simulink model "PFMODEL"  (R2023a)
settings: Solver=ode4  StartTime=0.0  StopTime=10  FixedStep=10e-6  RelTol=1e-3
libraries: spsPower3phInstantaneousLib x1, spsThreePhaseSeriesRLCLoadLib x1, spsThreePhaseVIMeasurementLib x1, spsThreePhaseSourceLib x1, sps_lib x1
settings Model: PacingRate=0.100000  Creator=KeronDenny  LastModifiedBy=KeronDenny

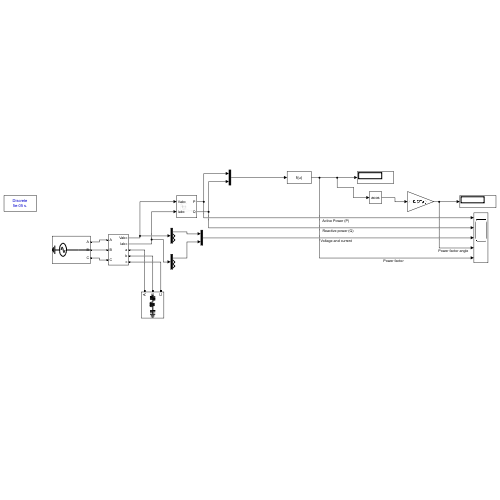
[thumbnail: Simulink's stored preview of the top-level diagram]
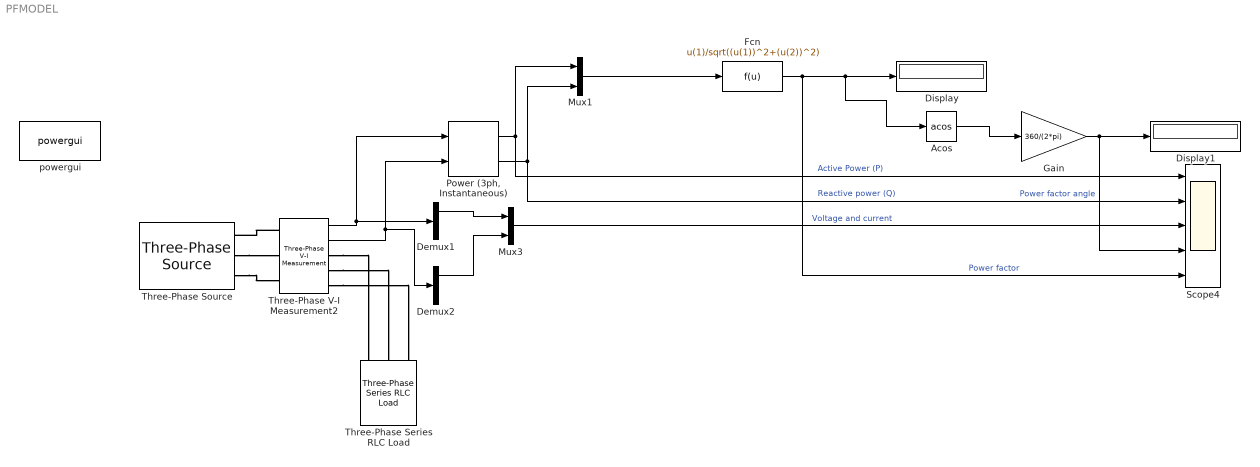
== system PFMODEL ==
  Acos : Trigonometry  Operator=acos
  Demux1 : Demux  Outputs=3
  Demux2 : Demux  Outputs=3
  Display : Display
  Display1 : Display
  Fcn : Fcn  Expr=u(1)/sqrt((u(1))^2+(u(2))^2)
  Gain : Gain  Gain=360/(2*pi)
  Mux1 : Mux  Inputs=2
  Mux3 : Mux  Inputs=2
  "Power (3ph, Instantaneous)" : spsPower3phInstantaneousLib/Power (3ph, Instantaneous)
  Scope4 : Scope  NumInputPorts=5
  Three-Phase Series RLC Load : spsThreePhaseSeriesRLCLoadLib/Three-Phase Series RLC Load  LConnTagsString=A|B|C  Configuration=Y (grounded)  NominalVoltage=400  Vabc=[1e3 1e3 1e3]  Vabcp=[1e3 1e3 1e3]  NominalFrequency=50  UnbalancedPower=off  ActivePower=40000  InductivePower=9012  CapacitivePower=35.92  Pabc=[10e3 9e3 11e3]  QLabc=[100 90 110]  QCabc=[100 90 110]  Pabcp=[10e3 9e3 11e3]  QLabcp=[100 90 110]  QCabcp=[100 90 110]  Measurements=None  LoadType=constant Z
  Three-Phase V-I Measurement2 : spsThreePhaseVIMeasurementLib/Three-Phase V-I Measurement  VoltageMeasurement=phase-to-ground  SetLabelV=off  LabelV=Vabc  Vpu=off  VpuLL=off  CurrentMeasurement=yes  SetLabelI=off  LabelI=Iabc  Ipu=off  Pbase=100e6  Vbase=500e3  OutputType=Complex  PhasorSimulation=off  PSBequivalent=0
  Three-Phase Source : spsThreePhaseSourceLib/Three-Phase Source  InternalConnection=Yg  VoltagePhases=off  Voltage=400  PhaseAngle=0  Voltage_phases=[25e3 25e3 25e3]/sqrt(3)  PhaseAngles_phases=[0 -120 +120]  Frequency=50  NonIdealSource=off  SpecifyImpedance=off  Resistance=0.8929  Inductance=16.58e-3  ShortCircuitLevel=100e6  BaseVoltage=25e3  XRratio=7  BusType=swing  Pref=10e3  Qref=0  Prefabc=[10e3, 10e3, 10e3]  Qrefabc=[0, 0, 0]  Qmin=-inf  Qmax=inf
  powergui : sps_lib/powergui  Priority=1  SimulationMode=Discrete  SampleTime=50e-6  frequency=60  Iterations=50  frequencyindice=50  Pbase=100e6  ErrMax=1e-4  UnitsV=kV  UnitsW=MW  buscounter=0  FunctionMessages=off  echomessages=off  EnableUseOfTLC=off  CurrentSourceSwitches=off  DisableSnubberDevices=off  DisableRonSwitches=off  DisableVfSwitches=off  DisplayEquations=off  AutomaticDiscreteSolvers=off  SolverType=Tustin/Backward Euler (TBE)  Interpol=off  ExternalGateDelay=off  methode=off  Ts=100  x0status=blocks  SPID=on  SwTol=0  HookPort=off  NonlinearTolerance=1e-4  nMaxIteration=100  ContinueOnMaxIteration=off  RestoreLinks=warning  ResistiveCurrentMeasurement=off  Frange=[0:2:500]  Ylog=off  Xlog=on  ShowGrid=off  save=off  variable=ZData  structure=0  ZoomFFT=off  StartTime=0.0  cycles=1  DisplayStyle=1  fundamental=60  FreqAxis=off  MaxFrequency=1000  frequencyindicesteady=1  RmsSteady=1  display=off
  wires:
  Demux1/1 -> Mux3/1
  Demux2/1 -> Mux3/2
  Three-Phase V-I Measurement2/1 -> Demux1/1, "Power (3ph, Instantaneous)"/1
  Mux3/1 -> Scope4/3  "Voltage and current"
  "Power (3ph, Instantaneous)"/1 -> Mux1/1, Scope4/1  "Active Power (P)"
  "Power (3ph, Instantaneous)"/2 -> Mux1/2, Scope4/2  "Reactive power (Q)"
  Three-Phase V-I Measurement2/2 -> Demux2/1, "Power (3ph, Instantaneous)"/2
  Mux1/1 -> Fcn/1
  Fcn/1 -> Scope4/5, Acos/1, Display/1  "Power factor"
  Acos/1 -> Gain/1
  Gain/1 -> Scope4/4, Display1/1  "Power factor angle"
  connections:
  Three-Phase Source/RConn2 -- Three-Phase V-I Measurement2/LConn2
  Three-Phase V-I Measurement2/LConn1 -- Three-Phase Source/RConn1
  Three-Phase V-I Measurement2/RConn3 -- Three-Phase Series RLC Load/LConn3
  Three-Phase Source/RConn3 -- Three-Phase V-I Measurement2/LConn3
  Three-Phase V-I Measurement2/RConn1 -- Three-Phase Series RLC Load/LConn1
  Three-Phase V-I Measurement2/RConn2 -- Three-Phase Series RLC Load/LConn2
